simulink subsystem "A312"  (R2022b)
settings: Solver=VariableStepAuto  StartTime=0.0  StopTime=10.0  RelTol=1e-3
settings Model: Creator=brent  LastModifiedBy=virgi

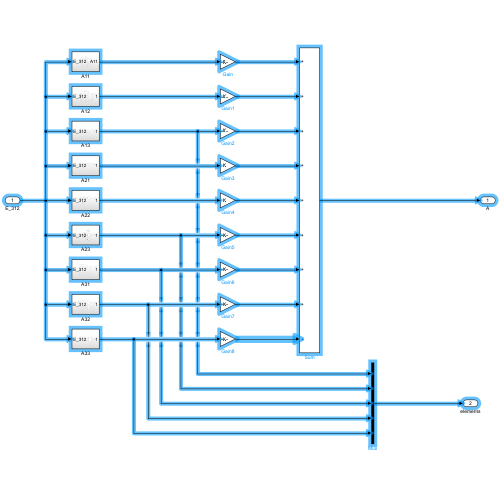
[thumbnail: Simulink's stored preview of the top-level diagram]
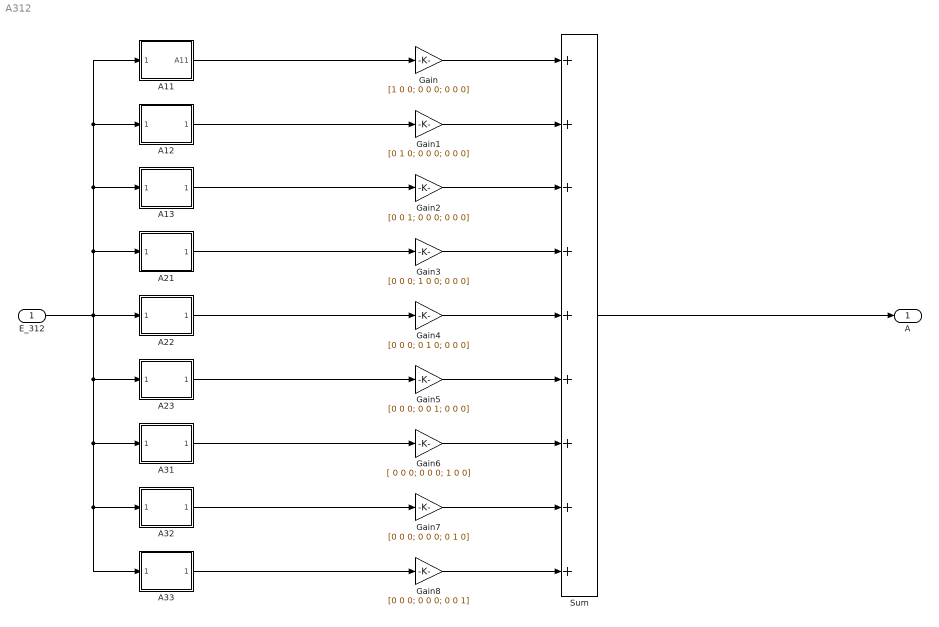
== system A312 ==
  E_312 : Inport
  A11 : Subsystem
  A12 : Subsystem
  A13 : Subsystem
  A21 : Subsystem
  A22 : Subsystem
  A23 : Subsystem
  A31 : Subsystem
  A32 : Subsystem
  A33 : Subsystem
  Gain : Gain  Gain=[1 0 0; 0 0 0; 0 0 0]
  Gain1 : Gain  Gain=[0 1 0; 0 0 0; 0 0 0]
  Gain2 : Gain  Gain=[0 0 1; 0 0 0; 0 0 0]
  Gain3 : Gain  Gain=[0 0 0; 1 0 0; 0 0 0]
  Gain4 : Gain  Gain=[0 0 0; 0 1 0; 0 0 0]
  Gain5 : Gain  Gain=[0 0 0; 0 0 1; 0 0 0]
  Gain6 : Gain  Gain=[ 0 0 0; 0 0 0; 1 0 0]
  Gain7 : Gain  Gain=[0 0 0; 0 0 0; 0 1 0]
  Gain8 : Gain  Gain=[0 0 0; 0 0 0; 0 0 1]
  Sum : Sum  Inputs=+++++++++
  A : Outport
  wires:
  Gain1/1 -> Sum/2
  Gain7/1 -> Sum/8
  Gain6/1 -> Sum/7
  Gain4/1 -> Sum/5
  A21/1(Out1) -> Gain3/1
  Gain/1 -> Sum/1
  A32/1(Out1) -> Gain7/1
  A22/1(Out1) -> Gain4/1
  Gain2/1 -> Sum/3
  A31/1(Out1) -> Gain6/1
  Sum/1 -> A/1
  E_312/1 -> A33/1(E_312), A32/1(E_312), A31/1(E_312), A23/1(E_312), A22/1(E_312), A12/1(E_312), A11/1(E_312), A13/1(E_312), A21/1(E_312)
  A11/1(A11) -> Gain/1
  A13/1(Out1) -> Gain2/1
  A33/1(Out1) -> Gain8/1
  A23/1(Out1) -> Gain5/1
  Gain3/1 -> Sum/4
  A12/1(Out1) -> Gain1/1
  Gain5/1 -> Sum/6
  Gain8/1 -> Sum/9

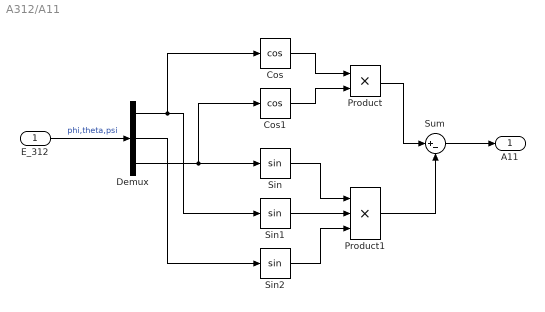
== system A312/A11 ==
  E_312 : Inport
  Cos : Trigonometry  Operator=cos
  Cos1 : Trigonometry  Operator=cos
  Demux : Demux  Outputs=3
  Product : Product
  Product1 : Product  Inputs=3
  Sin : Trigonometry
  Sin1 : Trigonometry
  Sin2 : Trigonometry
  Sum : Sum  Inputs=|+-
  A11 : Outport
  wires:
  E_312/1 -> Demux/1  "phi,theta,psi"
  Demux/3 -> Sin/1, Cos1/1
  Demux/1 -> Sin1/1, Cos/1
  Demux/2 -> Sin2/1
  Cos/1 -> Product/1
  Cos1/1 -> Product/2
  Sin1/1 -> Product1/2
  Sin2/1 -> Product1/3
  Sin/1 -> Product1/1
  Product/1 -> Sum/1
  Product1/1 -> Sum/2
  Sum/1 -> A11/1

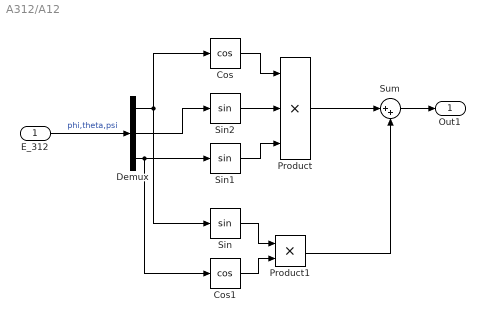
== system A312/A12 ==
  E_312 : Inport
  Cos : Trigonometry  Operator=cos
  Cos1 : Trigonometry  Operator=cos
  Demux : Demux  Outputs=3
  Product : Product  Inputs=3
  Product1 : Product
  Sin : Trigonometry
  Sin1 : Trigonometry
  Sin2 : Trigonometry
  Sum : Sum  Inputs=|++
  Out1 : Outport
  wires:
  E_312/1 -> Demux/1  "phi,theta,psi"
  Demux/3 -> Sin1/1, Cos1/1
  Demux/1 -> Sin/1, Cos/1
  Demux/2 -> Sin2/1
  Sin/1 -> Product1/1
  Cos1/1 -> Product1/2
  Sin2/1 -> Product/2
  Cos/1 -> Product/1
  Sin1/1 -> Product/3
  Sum/1 -> Out1/1
  Product/1 -> Sum/1
  Product1/1 -> Sum/2

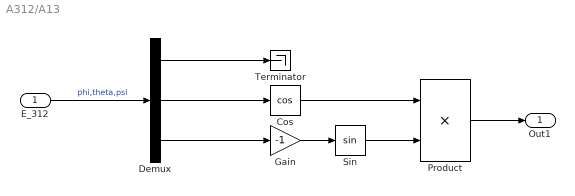
== system A312/A13 ==
  E_312 : Inport
  Cos : Trigonometry  Operator=cos
  Demux : Demux  Outputs=3
  Gain : Gain  Gain=-1
  Product : Product
  Sin : Trigonometry
  Terminator : Terminator
  Out1 : Outport
  wires:
  E_312/1 -> Demux/1  "phi,theta,psi"
  Gain/1 -> Sin/1
  Cos/1 -> Product/1
  Demux/2 -> Cos/1
  Demux/3 -> Gain/1
  Sin/1 -> Product/2
  Product/1 -> Out1/1
  Demux/1 -> Terminator/1

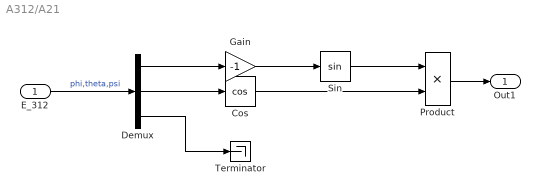
== system A312/A21 ==
  E_312 : Inport
  Cos : Trigonometry  Operator=cos
  Demux : Demux  Outputs=3
  Gain : Gain  Gain=-1
  Product : Product
  Sin : Trigonometry
  Terminator : Terminator
  Out1 : Outport
  wires:
  E_312/1 -> Demux/1  "phi,theta,psi"
  Demux/1 -> Gain/1
  Gain/1 -> Sin/1
  Sin/1 -> Product/1
  Demux/2 -> Cos/1
  Cos/1 -> Product/2
  Product/1 -> Out1/1
  Demux/3 -> Terminator/1

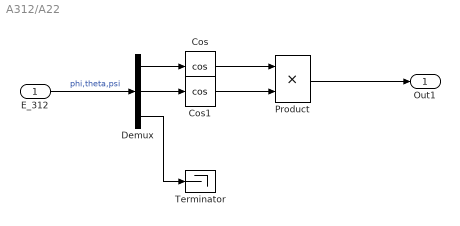
== system A312/A22 ==
  E_312 : Inport
  Cos : Trigonometry  Operator=cos
  Cos1 : Trigonometry  Operator=cos
  Demux : Demux  Outputs=3
  Product : Product
  Terminator : Terminator
  Out1 : Outport
  wires:
  E_312/1 -> Demux/1  "phi,theta,psi"
  Demux/1 -> Cos/1
  Demux/2 -> Cos1/1
  Cos1/1 -> Product/2
  Cos/1 -> Product/1
  Product/1 -> Out1/1
  Demux/3 -> Terminator/1

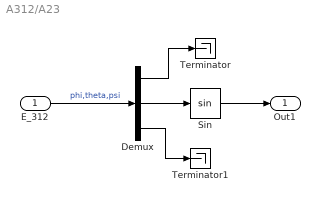
== system A312/A23 ==
  E_312 : Inport
  Demux : Demux  Outputs=3
  Sin : Trigonometry
  Terminator : Terminator
  Terminator1 : Terminator
  Out1 : Outport
  wires:
  E_312/1 -> Demux/1  "phi,theta,psi"
  Demux/2 -> Sin/1
  Sin/1 -> Out1/1
  Demux/3 -> Terminator1/1
  Demux/1 -> Terminator/1

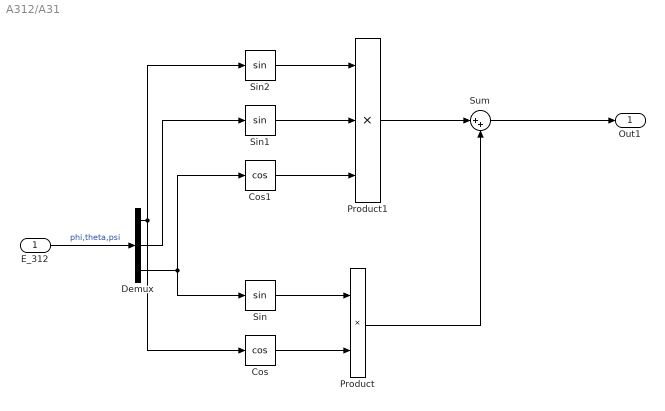
== system A312/A31 ==
  E_312 : Inport
  Cos : Trigonometry  Operator=cos
  Cos1 : Trigonometry  Operator=cos
  Demux : Demux  Outputs=3
  Product : Product
  Product1 : Product  Inputs=3
  Sin : Trigonometry
  Sin1 : Trigonometry
  Sin2 : Trigonometry
  Sum : Sum  Inputs=|++
  Out1 : Outport
  wires:
  E_312/1 -> Demux/1  "phi,theta,psi"
  Demux/3 -> Sin/1, Cos1/1
  Cos/1 -> Product/2
  Sin/1 -> Product/1
  Demux/1 -> Sin2/1, Cos/1
  Demux/2 -> Sin1/1
  Sin2/1 -> Product1/1
  Sin1/1 -> Product1/2
  Cos1/1 -> Product1/3
  Sum/1 -> Out1/1
  Product1/1 -> Sum/1
  Product/1 -> Sum/2

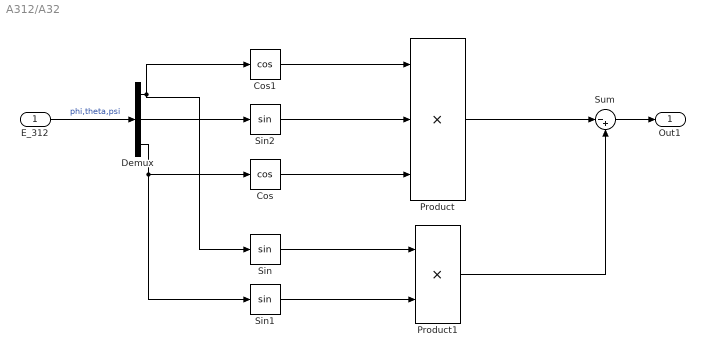
== system A312/A32 ==
  E_312 : Inport
  Cos : Trigonometry  Operator=cos
  Cos1 : Trigonometry  Operator=cos
  Demux : Demux  Outputs=3
  Product : Product  Inputs=3
  Product1 : Product
  Sin : Trigonometry
  Sin1 : Trigonometry
  Sin2 : Trigonometry
  Sum : Sum  Inputs=|-+
  Out1 : Outport
  wires:
  E_312/1 -> Demux/1  "phi,theta,psi"
  Demux/1 -> Cos1/1, Sin/1
  Demux/3 -> Cos/1, Sin1/1
  Demux/2 -> Sin2/1
  Cos/1 -> Product/3
  Sin2/1 -> Product/2
  Cos1/1 -> Product/1
  Sin1/1 -> Product1/2
  Sin/1 -> Product1/1
  Product/1 -> Sum/1
  Product1/1 -> Sum/2
  Sum/1 -> Out1/1

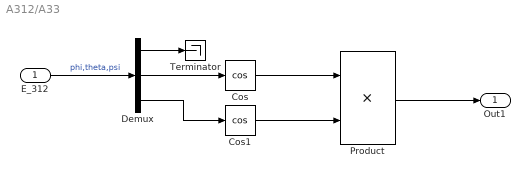
== system A312/A33 ==
  E_312 : Inport
  Cos : Trigonometry  Operator=cos
  Cos1 : Trigonometry  Operator=cos
  Demux : Demux  Outputs=3
  Product : Product
  Terminator : Terminator
  Out1 : Outport
  wires:
  E_312/1 -> Demux/1  "phi,theta,psi"
  Demux/2 -> Cos/1
  Demux/3 -> Cos1/1
  Cos1/1 -> Product/2
  Product/1 -> Out1/1
  Cos/1 -> Product/1
  Demux/1 -> Terminator/1
